simulink library "halout"  (R2021b)
settings: Solver=VariableStepAuto  StartTime=0.0  StopTime=10.0  RelTol=1e-3
undefined symbols (not defined in the file): C_TASK_5MS_S, FALSE, KHAL_CAN1FDAPS3E2E_flg, KHAL_CAN1FDAPS3TxReq_flg, KHAL_CAN1FDVCU2E2E_flg, KHAL_CAN1FDVCU2TxReq_flg, KHAL_CAN1FDVCU3E2E_flg, KHAL_CAN1FDVCU3TxReq_flg, KHAL_CAN1TxReq_flg, KHAL_CAN2TxReq_flg, KHAL_CAN3FDVCU1TxReq_flg, KHAL_CAN3FDVCU2E2E_flg, KHAL_CAN3FDVCU2TxReq_flg, KHAL_CAN3TxReq_flg, KHAL_CAN4FDVCU1E2E_flg, KHAL_CAN4FDVCU1TxReq_flg, KHAL_CAN4TxReq_flg, KHAL_CAN5TxReq_flg, ONE_INT, TRUE, ZERO_INT
libraries: FVT_lib x383, simulink x179
(part 7 of 20)

== system halout/HAL_OUT/CAN3/FD_THCM2_0x186 ==
  BSCP_outputs : Inport  OutDataTypeStr=Bus: BSCP_outputs
  BOUTP_outputs : Inport  Port=2  OutDataTypeStr=Bus: BOUTP_outputs
  ACSubMode : Subsystem
  APTCActFrRiPwr : Subsystem
  BatLoopActWtFlw : Subsystem
  CCUCbnPreACWkSts : Subsystem
  CCUCbnPreEstimdTi : Subsystem
  CCUCbnPreSts : Subsystem
  CCUHiVoltageReq : Subsystem
  CoolgFanActDuty : Subsystem
  DeiceModReq : Subsystem
  FDBlowerCmd : Subsystem
  FDCompCmd : Subsystem
  FDEWP1Cmd : Subsystem
  FDEWP2Cmd : Subsystem
  FDEWP3Cmd : Subsystem
  FDEXV1Cmd : Subsystem
  FDEXV2Cmd : Subsystem
  FDFWVCmd : Subsystem
  FDFrLeAPTCHeatPwrCmd : Subsystem
  FDFrRiAPTCHeatPwrCmd : Subsystem
  FDFrWPTCHeatPwrCmd : Subsystem
  FDRrAPTCHeatPwrCmd : Subsystem
  FDSOTXVCmd : Subsystem
  FDSOV1Cmd : Subsystem
  FDSOV2Cmd : Subsystem
  FDSOV3Cmd : Subsystem
  FDTWVCmd : Subsystem
  Ground{,1..6} (7 alike) : Ground
  bus_creator : BusCreator  Inputs=26  OutDataTypeStr=Bus: DT_CAN3_SG_FD_THCM2  NonVirtualBus=on
  bus_selector : BusSelector  OutputSignals=VOUTP_ACSubMode_enum
  bus_selector1 : BusSelector  OutputSignals=VOUTP_CoolgFanActDuty_pct
  bus_selector10 : BusSelector  OutputSignals=VOUTP_FDFrLeAPTCHeatPwrCmd_W
  bus_selector11 : BusSelector  OutputSignals=VOUTP_FDFrRiAPTCHeatPwrCmd_W
  bus_selector12 : BusSelector  OutputSignals=VOUTP_FDFrWPTCHeatPwrCmd_W
  bus_selector13 : BusSelector  OutputSignals=VOUTP_FDRrAPTCHeatPwrCmd_W
  bus_selector14 : BusSelector  OutputSignals=VOUTP_FDSOTXVCmd_flg
  bus_selector15 : BusSelector  OutputSignals=VOUTP_FDSOV1Cmd_flg
  bus_selector16 : BusSelector  OutputSignals=VOUTP_FDSOV2Cmd_flg
  bus_selector17 : BusSelector  OutputSignals=VOUTP_FDSOV3Cmd_flg
  bus_selector18 : BusSelector  OutputSignals=VOUTP_FDTWVCmd_pct
  bus_selector2 : BusSelector  OutputSignals=VOUTP_FDBlowerCmd_pct
  bus_selector3 : BusSelector  OutputSignals=VOUTP_FDCompCmd_rpm
  bus_selector4 : BusSelector  OutputSignals=VOUTP_FDEWP1Cmd_enum
  bus_selector5 : BusSelector  OutputSignals=VOUTP_FDEWP2Cmd_enum
  bus_selector6 : BusSelector  OutputSignals=VOUTP_FDEWP3Cmd_enum
  bus_selector7 : BusSelector  OutputSignals=VOUTP_FDEXV1Cmd_step
  bus_selector8 : BusSelector  OutputSignals=VOUTP_FDEXV2Cmd_step
  bus_selector9 : BusSelector  OutputSignals=VOUTP_FDFWVCmd_flg
  FD_THCM2 : Outport
  wires:
  BSCP_outputs/1 -> [BSCP_outputs]
  BOUTP_outputs/1 -> [BOUTP_outputs]
  [CAN3_ACSubMode] -> bus_creator/1  "CAN3_ACSubMode"
  [CAN3_APTC_ActFrRiPwr] -> bus_creator/2  "CAN3_APTC_ActFrRiPwr"
  [CAN3_BatLoopActWtFlw] -> bus_creator/3  "CAN3_BatLoopActWtFlw"
  [CAN3_CCU_CbnPreACWkSts] -> bus_creator/4  "CAN3_CCU_CbnPreACWkSts"
  [CAN3_CCU_CbnPreEstimdTi] -> bus_creator/5  "CAN3_CCU_CbnPreEstimdTi"
  [CAN3_CCU_CbnPreSts] -> bus_creator/6  "CAN3_CCU_CbnPreSts"
  [CAN3_CCU_HiVoltageReq] -> bus_creator/7  "CAN3_CCU_HiVoltageReq"
  [CAN3_CoolgFanActDuty] -> bus_creator/8  "CAN3_CoolgFanActDuty"
  [CAN3_DeiceModReq] -> bus_creator/9  "CAN3_DeiceModReq"
  [CAN3_FD_Blower_Cmd] -> bus_creator/10  "CAN3_FD_Blower_Cmd"
  [CAN3_FD_Comp_Cmd] -> bus_creator/11  "CAN3_FD_Comp_Cmd"
  [CAN3_FD_EWP1_Cmd] -> bus_creator/12  "CAN3_FD_EWP1_Cmd"
  [CAN3_FD_EWP2_Cmd] -> bus_creator/13  "CAN3_FD_EWP2_Cmd"
  [CAN3_FD_EWP3_Cmd] -> bus_creator/14  "CAN3_FD_EWP3_Cmd"
  [CAN3_FD_EXV1_Cmd] -> bus_creator/15  "CAN3_FD_EXV1_Cmd"
  [CAN3_FD_EXV2_Cmd] -> bus_creator/16  "CAN3_FD_EXV2_Cmd"
  [CAN3_FD_FWV_Cmd] -> bus_creator/17  "CAN3_FD_FWV_Cmd"
  [CAN3_FD_FrLeAPTCHeatPwr_Cmd] -> bus_creator/18  "CAN3_FD_FrLeAPTCHeatPwr_Cmd"
  [CAN3_FD_FrRiAPTCHeatPwr_Cmd] -> bus_creator/19  "CAN3_FD_FrRiAPTCHeatPwr_Cmd"
  [CAN3_FD_FrWPTCHeatPwr_Cmd] -> bus_creator/20  "CAN3_FD_FrWPTCHeatPwr_Cmd"
  [CAN3_FD_RrAPTCHeatPwr_Cmd] -> bus_creator/21  "CAN3_FD_RrAPTCHeatPwr_Cmd"
  [CAN3_FD_SOTXV_Cmd] -> bus_creator/22  "CAN3_FD_SOTXV_Cmd"
  [CAN3_FD_SOV1_Cmd] -> bus_creator/23  "CAN3_FD_SOV1_Cmd"
  [CAN3_FD_SOV2_Cmd] -> bus_creator/24  "CAN3_FD_SOV2_Cmd"
  [CAN3_FD_SOV3_Cmd] -> bus_creator/25  "CAN3_FD_SOV3_Cmd"
  [CAN3_FD_TWV_Cmd] -> bus_creator/26  "CAN3_FD_TWV_Cmd"
  bus_creator/1 -> FD_THCM2/1
  ACSubMode/1(CAN3_ACSubMode) -> [CAN3_ACSubMode]
  APTCActFrRiPwr/1(CAN3_APTC_ActFrRiPwr) -> [CAN3_APTC_ActFrRiPwr]
  BatLoopActWtFlw/1(CAN3_BatLoopActWtFlw) -> [CAN3_BatLoopActWtFlw]
  CCUCbnPreACWkSts/1(CAN3_CCU_CbnPreACWkSts) -> [CAN3_CCU_CbnPreACWkSts]
  CCUCbnPreEstimdTi/1(CAN3_CCU_CbnPreEstimdTi) -> [CAN3_CCU_CbnPreEstimdTi]
  CCUCbnPreSts/1(CAN3_CCU_CbnPreSts) -> [CAN3_CCU_CbnPreSts]
  CCUHiVoltageReq/1(CAN3_CCU_HiVoltageReq) -> [CAN3_CCU_HiVoltageReq]
  CoolgFanActDuty/1(CAN3_CoolgFanActDuty) -> [CAN3_CoolgFanActDuty]
  DeiceModReq/1(CAN3_DeiceModReq) -> [CAN3_DeiceModReq]
  FDBlowerCmd/1(CAN3_FD_Blower_Cmd) -> [CAN3_FD_Blower_Cmd]
  FDCompCmd/1(CAN3_FD_Comp_Cmd) -> [CAN3_FD_Comp_Cmd]
  FDEWP1Cmd/1(CAN3_FD_EWP1_Cmd) -> [CAN3_FD_EWP1_Cmd]
  FDEWP2Cmd/1(CAN3_FD_EWP2_Cmd) -> [CAN3_FD_EWP2_Cmd]
  FDEWP3Cmd/1(CAN3_FD_EWP3_Cmd) -> [CAN3_FD_EWP3_Cmd]
  FDEXV1Cmd/1(CAN3_FD_EXV1_Cmd) -> [CAN3_FD_EXV1_Cmd]
  FDEXV2Cmd/1(CAN3_FD_EXV2_Cmd) -> [CAN3_FD_EXV2_Cmd]
  FDFWVCmd/1(CAN3_FD_FWV_Cmd) -> [CAN3_FD_FWV_Cmd]
  FDFrLeAPTCHeatPwrCmd/1(CAN3_FD_FrLeAPTCHeatPwr_Cmd) -> [CAN3_FD_FrLeAPTCHeatPwr_Cmd]
  FDFrRiAPTCHeatPwrCmd/1(CAN3_FD_FrRiAPTCHeatPwr_Cmd) -> [CAN3_FD_FrRiAPTCHeatPwr_Cmd]
  FDFrWPTCHeatPwrCmd/1(CAN3_FD_FrWPTCHeatPwr_Cmd) -> [CAN3_FD_FrWPTCHeatPwr_Cmd]
  FDRrAPTCHeatPwrCmd/1(CAN3_FD_RrAPTCHeatPwr_Cmd) -> [CAN3_FD_RrAPTCHeatPwr_Cmd]
  FDSOTXVCmd/1(CAN3_FD_SOTXV_Cmd) -> [CAN3_FD_SOTXV_Cmd]
  FDSOV1Cmd/1(CAN3_FD_SOV1_Cmd) -> [CAN3_FD_SOV1_Cmd]
  FDSOV2Cmd/1(CAN3_FD_SOV2_Cmd) -> [CAN3_FD_SOV2_Cmd]
  FDSOV3Cmd/1(CAN3_FD_SOV3_Cmd) -> [CAN3_FD_SOV3_Cmd]
  FDTWVCmd/1(CAN3_FD_TWV_Cmd) -> [CAN3_FD_TWV_Cmd]
  bus_selector/1 -> ACSubMode/1(ACSubMode)  "<VOUTP_ACSubMode_enum>"
  [BOUTP_outputs] -> bus_selector/1
  Ground/1 -> APTCActFrRiPwr/1(APTCActFrRiPwr)
  Ground1/1 -> BatLoopActWtFlw/1(BatLoopActWtFlw)
  Ground2/1 -> CCUCbnPreACWkSts/1(CCUCbnPreACWkSts)
  Ground3/1 -> CCUCbnPreEstimdTi/1(CCUCbnPreEstimdTi)
  Ground4/1 -> CCUCbnPreSts/1(CCUCbnPreSts)
  Ground5/1 -> CCUHiVoltageReq/1(CCUHiVoltageReq)
  bus_selector1/1 -> CoolgFanActDuty/1(CoolgFanActDuty)  "<VOUTP_CoolgFanActDuty_pct>"
  [BOUTP_outputs] -> bus_selector1/1
  Ground6/1 -> DeiceModReq/1(DeiceModReq)
  bus_selector2/1 -> FDBlowerCmd/1(FDBlowerCmd)  "<VOUTP_FDBlowerCmd_pct>"
  [BOUTP_outputs] -> bus_selector2/1
  bus_selector3/1 -> FDCompCmd/1(FDCompCmd)  "<VOUTP_FDCompCmd_rpm>"
  [BOUTP_outputs] -> bus_selector3/1
  bus_selector4/1 -> FDEWP1Cmd/1(FDEWP1Cmd)  "<VOUTP_FDEWP1Cmd_enum>"
  [BOUTP_outputs] -> bus_selector4/1
  bus_selector5/1 -> FDEWP2Cmd/1(FDEWP2Cmd)  "<VOUTP_FDEWP2Cmd_enum>"
  [BOUTP_outputs] -> bus_selector5/1
  bus_selector6/1 -> FDEWP3Cmd/1(FDEWP3Cmd)  "<VOUTP_FDEWP3Cmd_enum>"
  [BOUTP_outputs] -> bus_selector6/1
  bus_selector7/1 -> FDEXV1Cmd/1(FDEXV1Cmd)  "<VOUTP_FDEXV1Cmd_step>"
  [BOUTP_outputs] -> bus_selector7/1
  bus_selector8/1 -> FDEXV2Cmd/1(FDEXV2Cmd)  "<VOUTP_FDEXV2Cmd_step>"
  [BOUTP_outputs] -> bus_selector8/1
  bus_selector9/1 -> FDFWVCmd/1(FDFWVCmd)  "<VOUTP_FDFWVCmd_flg>"
  [BOUTP_outputs] -> bus_selector9/1
  bus_selector10/1 -> FDFrLeAPTCHeatPwrCmd/1(FDFrLeAPTCHeatPwrCmd)  "<VOUTP_FDFrLeAPTCHeatPwrCmd_W>"
  [BOUTP_outputs] -> bus_selector10/1
  bus_selector11/1 -> FDFrRiAPTCHeatPwrCmd/1(FDFrRiAPTCHeatPwrCmd)  "<VOUTP_FDFrRiAPTCHeatPwrCmd_W>"
  [BOUTP_outputs] -> bus_selector11/1
  bus_selector12/1 -> FDFrWPTCHeatPwrCmd/1(FDFrWPTCHeatPwrCmd)  "<VOUTP_FDFrWPTCHeatPwrCmd_W>"
  [BOUTP_outputs] -> bus_selector12/1
  bus_selector13/1 -> FDRrAPTCHeatPwrCmd/1(FDRrAPTCHeatPwrCmd)  "<VOUTP_FDRrAPTCHeatPwrCmd_W>"
  [BOUTP_outputs] -> bus_selector13/1
  bus_selector14/1 -> FDSOTXVCmd/1(FDSOTXVCmd)  "<VOUTP_FDSOTXVCmd_flg>"
  [BOUTP_outputs] -> bus_selector14/1
  bus_selector15/1 -> FDSOV1Cmd/1(FDSOV1Cmd)  "<VOUTP_FDSOV1Cmd_flg>"
  [BOUTP_outputs] -> bus_selector15/1
  bus_selector16/1 -> FDSOV2Cmd/1(FDSOV2Cmd)  "<VOUTP_FDSOV2Cmd_flg>"
  [BOUTP_outputs] -> bus_selector16/1
  bus_selector17/1 -> FDSOV3Cmd/1(FDSOV3Cmd)  "<VOUTP_FDSOV3Cmd_flg>"
  [BOUTP_outputs] -> bus_selector17/1
  bus_selector18/1 -> FDTWVCmd/1(FDTWVCmd)  "<VOUTP_FDTWVCmd_pct>"
  [BOUTP_outputs] -> bus_selector18/1

== system halout/HAL_OUT/CAN3/FD_V2L1_0x374 ==
  BSCP_outputs : Inport  OutDataTypeStr=Bus: BSCP_outputs
  BOUTP_outputs : Inport  Port=2  OutDataTypeStr=Bus: BOUTP_outputs
  Ground : Ground
  ReqOBCV2LEna : Subsystem
  ReqV2LIVIPopup : Subsystem
  ReqV2LSwOn : Subsystem
  bus_creator : BusCreator  Inputs=3  OutDataTypeStr=Bus: DT_CAN3_SG_FD_V2L1  NonVirtualBus=on
  bus_selector : BusSelector  OutputSignals=VOUTP_ReqOBCV2LEna_enum
  bus_selector1 : BusSelector  OutputSignals=VOUTP_ReqV2LIVIPopup_enum
  FD_V2L1 : Outport
  wires:
  BSCP_outputs/1 -> [BSCP_outputs]
  BOUTP_outputs/1 -> [BOUTP_outputs]
  [CAN3_Req_OBCV2LEna] -> bus_creator/1  "CAN3_Req_OBCV2LEna"
  [CAN3_Req_V2LSwOn] -> bus_creator/2  "CAN3_Req_V2LSwOn"
  [CAN3_Req_V2L_IVI_Popup] -> bus_creator/3  "CAN3_Req_V2L_IVI_Popup"
  bus_creator/1 -> FD_V2L1/1
  ReqOBCV2LEna/1(CAN3_Req_OBCV2LEna) -> [CAN3_Req_OBCV2LEna]
  ReqV2LSwOn/1(CAN3_Req_V2LSwOn) -> [CAN3_Req_V2LSwOn]
  ReqV2LIVIPopup/1(CAN3_Req_V2L_IVI_Popup) -> [CAN3_Req_V2L_IVI_Popup]
  bus_selector/1 -> ReqOBCV2LEna/1(ReqOBCV2LEna)  "<VOUTP_ReqOBCV2LEna_enum>"
  [BOUTP_outputs] -> bus_selector/1
  Ground/1 -> ReqV2LSwOn/1(ReqV2LSwOn)
  bus_selector1/1 -> ReqV2LIVIPopup/1(ReqV2LIVIPopup)  "<VOUTP_ReqV2LIVIPopup_enum>"
  [BOUTP_outputs] -> bus_selector1/1

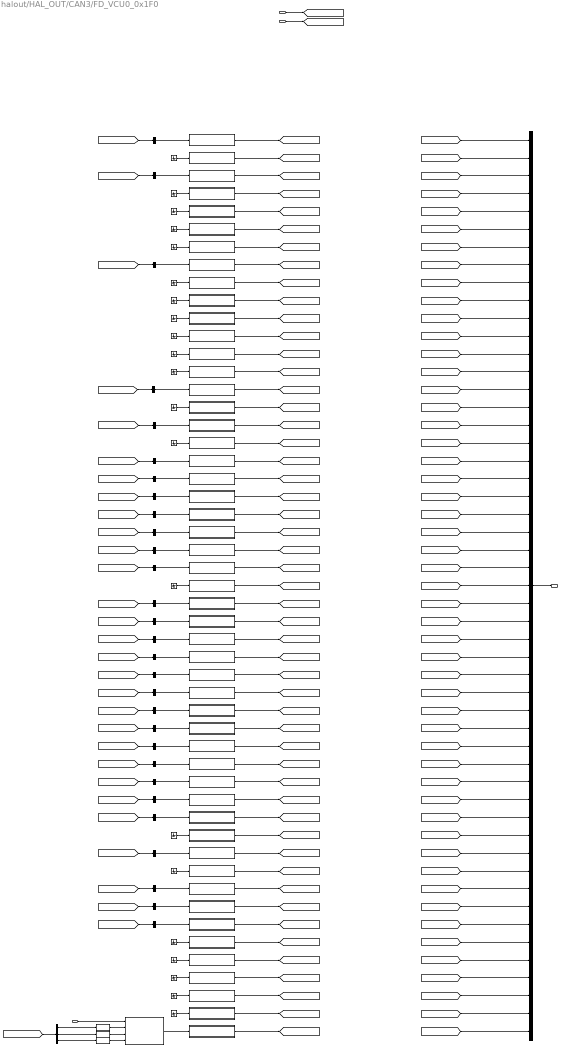
== system halout/HAL_OUT/CAN3/FD_VCU0_0x1F0 ==
  BSCP_outputs : Inport  OutDataTypeStr=Bus: BSCP_outputs
  BOUTP_outputs : Inport  Port=2  OutDataTypeStr=Bus: BOUTP_outputs
  s8_AcoreReadyToSleep : Inport  Port=3
  Data Type Conversion : DataTypeConversion  OutDataTypeStr=uint8
  Data Type Conversion1 : DataTypeConversion  OutDataTypeStr=uint8
  Data Type Conversion2 : DataTypeConversion  OutDataTypeStr=uint8
  EVCCAplusPwrUpReq : Subsystem
  FDADC12VDet : Subsystem
  FDADC12VDetAvg : Subsystem
  FDCVCUActMaxSlideRateSta : Subsystem
  FDCVCUAllowMovThdOTASta : Subsystem
  FDCVCUDTCCarouselSta : Subsystem
  FDCVCUForcePCmd : Subsystem
  FDCVCUPwrReqOTASta : Subsystem
  FDCVCURWDRDCActiveSta : Subsystem
  FDCVCURegenTqLimitEnSta : Subsystem
  FDCVCUSlideRegenLimTqSta : Subsystem
  FDCVCUVehActSpdSta : Subsystem
  FDCVCUVehMalfunLevelSta : Subsystem
  FDCVMCActStESCYawSta : Subsystem
  FDCVMCAntiSpdLimEnSta : Subsystem
  FDCVMCLongAccSta : Subsystem
  FrTqSource : Subsystem
  Ground{,1..10,12..21} (21 alike) : Ground
  HVRlyOpFail : Subsystem
  HVTHCMSysAvail : Subsystem
  LVBattChrgtimeAct : Subsystem
  LVBattVoltSta : Subsystem
  LVChrgHoldTAct : Subsystem
  LVSilentChrgLv : Subsystem
  LVSilentChrgReq : Subsystem
  LVSilentChrgSta : Subsystem
  MCUActDisFail : Subsystem
  PMMAllowECUSleep : Subsystem
  PowerDownFault : Subsystem
  PowerDownState : Subsystem
  PowerUpFault : Subsystem
  PowerUpState : Subsystem
  PwrDownReq : Subsystem
  PwrStaConstraint : Subsystem
  PwrStaONTOIVIPopReq : Subsystem
  PwrStaONTOIVIPopT : Subsystem
  PwrStaSelect : Subsystem
  PwrStaTOSta : Subsystem
  PwrUpReq : Subsystem
  RrTqSource : Subsystem
  SchedChgTOSta : Subsystem
  SilentChkAllowSleep : Subsystem
  Subsystem : Subsystem
  SysAllowReadySta : Subsystem
  SysPwrSta : Subsystem
  TCountSta : Subsystem
  TimerAllowSleep : Subsystem
  VCUBrkSWSta : Subsystem
  VCUFLDoorSta : Subsystem
  VCUFRDoorSta : Subsystem
  VCURLDoorSta : Subsystem
  VCURRDoorSta : Subsystem
  VehHVPwrAvail4THCM : Subsystem
  bus_creator : BusCreator  Inputs=51  OutDataTypeStr=Bus: DT_CAN3_SG_FD_VCU0  NonVirtualBus=on
  bus_selector : BusSelector  OutputSignals=VOUTP_EvccAplusPwrUpReq_flg
  bus_selector1 : BusSelector  OutputSignals=VOUTP_FDADC12VDetAvg_mV
  bus_selector10 : BusSelector  OutputSignals=VOUTP_LVSilentChrgSta_enum
  bus_selector11 : BusSelector  OutputSignals=VOUTP_PMMAllowECUSleep_flg
  bus_selector12 : BusSelector  OutputSignals=VOUTP_PowerDownFault_enum
  bus_selector13 : BusSelector  OutputSignals=VOUTP_PowerDownState_enum
  bus_selector14 : BusSelector  OutputSignals=VOUTP_PowerUpFault_enum
  bus_selector15 : BusSelector  OutputSignals=VOUTP_PowerUpState_enum
  bus_selector16 : BusSelector  OutputSignals=VOUTP_PwrDownReq_enum
  bus_selector17 : BusSelector  OutputSignals=VOUTP_PwrStaConstraint_enum
  bus_selector18 : BusSelector  OutputSignals=VOUTP_PwrStaONTOPopReq_flg
  bus_selector19 : BusSelector  OutputSignals=VOUTP_IVIPwrStaONTOPopT_s
  bus_selector2 : BusSelector  OutputSignals=VOUTP_PwrReq_OTA_enum
  bus_selector20 : BusSelector  OutputSignals=VOUTP_PwrStaSelect_enum
  bus_selector21 : BusSelector  OutputSignals=VOUTP_PwrStaTOSta_enum
  bus_selector22 : BusSelector  OutputSignals=VOUTP_PwrUpReq_enum
  bus_selector23 : BusSelector  OutputSignals=VOUTP_TqSourceRr_enum
  bus_selector24 : BusSelector  OutputSignals=VOUTP_SilentChkAllowSleep_flg
  bus_selector25 : BusSelector  OutputSignals=VOUTP_SysPowerMode_enum
  bus_selector26 : BusSelector  OutputSignals=VOUTP_TCountSta_enum
  bus_selector27 : BusSelector  OutputSignals=VOUTP_TimerAllowSleep_flg
  bus_selector28 : BusSelector  OutputSignals=VOUTP_CurrentNmState_enum,VOUTP_OTAPwrReqOFFChkSta_enum,VOUTP_OTAPwrReqStdChkSta_enum
  bus_selector29 : BusSelector  OutputSignals=VOUTP_ExtraMSACtrlSta_enum
  bus_selector3 : BusSelector  OutputSignals=VOUTP_TqSourceFr_enum
  bus_selector4 : BusSelector  OutputSignals=VOUTP_HVTHCMSysAvail_enum
  bus_selector5 : BusSelector  OutputSignals=VOUTP_LVBattChrgTimeCnt_s
  bus_selector6 : BusSelector  OutputSignals=VOUTP_LVBattVoltSta_enum
  bus_selector7 : BusSelector  OutputSignals=VOUTP_LVChrgHoldTtimer_s
  bus_selector8 : BusSelector  OutputSignals=VOUTP_LVSilentChrgLv_enum
  bus_selector9 : BusSelector  OutputSignals=VOUTP_LVSilentChrgReq_flg
  FD_VCU0 : Outport
  wires:
  BSCP_outputs/1 -> [BSCP_outputs]
  BOUTP_outputs/1 -> [BOUTP_outputs]
  [CAN3_EVCCAplusPwrUpReq] -> bus_creator/1  "CAN3_EVCCAplusPwrUpReq"
  [CAN3_FDADC12VDet] -> bus_creator/2  "CAN3_FDADC12VDet"
  [CAN3_FDADC12VDetAvg] -> bus_creator/3  "CAN3_FDADC12VDetAvg"
  [CAN3_FDC_VCU_ActMaxSlideRate_Sta] -> bus_creator/4  "CAN3_FDC_VCU_ActMaxSlideRate_Sta"
  [CAN3_FDC_VCU_AllowMovThd_OTA_Sta] -> bus_creator/5  "CAN3_FDC_VCU_AllowMovThd_OTA_Sta"
  [CAN3_FDC_VCU_DTCCarousel_Sta] -> bus_creator/6  "CAN3_FDC_VCU_DTCCarousel_Sta"
  [CAN3_FDC_VCU_ForceP_Cmd] -> bus_creator/7  "CAN3_FDC_VCU_ForceP_Cmd"
  [CAN3_FDC_VCU_PwrReq_OTA_Sta] -> bus_creator/8  "CAN3_FDC_VCU_PwrReq_OTA_Sta"
  [CAN3_FDC_VCU_RWDRDCActive_Sta] -> bus_creator/9  "CAN3_FDC_VCU_RWDRDCActive_Sta"
  [CAN3_FDC_VCU_RegenTqLimitEn_Sta] -> bus_creator/10  "CAN3_FDC_VCU_RegenTqLimitEn_Sta"
  [CAN3_FDC_VCU_SlideRegenLimTq_Sta] -> bus_creator/11  "CAN3_FDC_VCU_SlideRegenLimTq_Sta"
  [CAN3_FDC_VCU_VehActSpd_Sta] -> bus_creator/12  "CAN3_FDC_VCU_VehActSpd_Sta"
  [CAN3_FDC_VCU_VehMalfunLevel_Sta] -> bus_creator/13  "CAN3_FDC_VCU_VehMalfunLevel_Sta"
  [CAN3_FDC_VMC_ActStESCYaw_Sta] -> bus_creator/14  "CAN3_FDC_VMC_ActStESCYaw_Sta"
  [CAN3_FDC_VMC_AntiSpdLimEn_Sta] -> bus_creator/15  "CAN3_FDC_VMC_AntiSpdLimEn_Sta"
  [CAN3_FDC_VMC_LongAcc_Sta] -> bus_creator/16  "CAN3_FDC_VMC_LongAcc_Sta"
  [CAN3_Fr_TqSource] -> bus_creator/17  "CAN3_Fr_TqSource"
  [CAN3_HVRlyOpFail] -> bus_creator/18  "CAN3_HVRlyOpFail"
  [CAN3_HVTHCMSysAvail] -> bus_creator/19  "CAN3_HVTHCMSysAvail"
  [CAN3_LVBattChrgtimeAct] -> bus_creator/20  "CAN3_LVBattChrgtimeAct"
  [CAN3_LVBattVoltSta] -> bus_creator/21  "CAN3_LVBattVoltSta"
  [CAN3_LVChrgHoldTAct] -> bus_creator/22  "CAN3_LVChrgHoldTAct"
  [CAN3_LVSilentChrgLv] -> bus_creator/23  "CAN3_LVSilentChrgLv"
  [CAN3_LVSilentChrgReq] -> bus_creator/24  "CAN3_LVSilentChrgReq"
  [CAN3_LVSilentChrgSta] -> bus_creator/25  "CAN3_LVSilentChrgSta"
  [CAN3_MCUActDisFail] -> bus_creator/26  "CAN3_MCUActDisFail"
  [CAN3_PMMAllowECUSleep] -> bus_creator/27  "CAN3_PMMAllowECUSleep"
  [CAN3_PowerDownFault] -> bus_creator/28  "CAN3_PowerDownFault"
  [CAN3_PowerDownState] -> bus_creator/29  "CAN3_PowerDownState"
  [CAN3_PowerUpFault] -> bus_creator/30  "CAN3_PowerUpFault"
  [CAN3_PowerUpState] -> bus_creator/31  "CAN3_PowerUpState"
  [CAN3_PwrDownReq] -> bus_creator/32  "CAN3_PwrDownReq"
  [CAN3_PwrStaConstraint] -> bus_creator/33  "CAN3_PwrStaConstraint"
  [CAN3_PwrStaONTOIVIPopReq] -> bus_creator/34  "CAN3_PwrStaONTOIVIPopReq"
  [CAN3_PwrStaONTOIVIPopT] -> bus_creator/35  "CAN3_PwrStaONTOIVIPopT"
  [CAN3_PwrStaSelect] -> bus_creator/36  "CAN3_PwrStaSelect"
  [CAN3_PwrStaTOSta] -> bus_creator/37  "CAN3_PwrStaTOSta"
  [CAN3_PwrUpReq] -> bus_creator/38  "CAN3_PwrUpReq"
  [CAN3_Rr_TqSource] -> bus_creator/39  "CAN3_Rr_TqSource"
  [CAN3_SchedChgTOSta] -> bus_creator/40  "CAN3_SchedChgTOSta"
  [CAN3_SilentChkAllowSleep] -> bus_creator/41  "CAN3_SilentChkAllowSleep"
  [CAN3_SysAllowReadySta] -> bus_creator/42  "CAN3_SysAllowReadySta"
  [CAN3_SysPwrSta] -> bus_creator/43  "CAN3_SysPwrSta"
  [CAN3_TCountSta] -> bus_creator/44  "CAN3_TCountSta"
  [CAN3_TimerAllowSleep] -> bus_creator/45  "CAN3_TimerAllowSleep"
  [CAN3_VCUBrkSWSta] -> bus_creator/46  "CAN3_VCUBrkSWSta"
  [CAN3_VCUFLDoorSta] -> bus_creator/47  "CAN3_VCUFLDoorSta"
  [CAN3_VCUFRDoorSta] -> bus_creator/48  "CAN3_VCUFRDoorSta"
  [CAN3_VCURLDoorSta] -> bus_creator/49  "CAN3_VCURLDoorSta"
  [CAN3_VCURRDoorSta] -> bus_creator/50  "CAN3_VCURRDoorSta"
  [CAN3_VehHVPwrAvail4THCM] -> bus_creator/51  "CAN3_VehHVPwrAvail4THCM"
  bus_creator/1 -> FD_VCU0/1
  EVCCAplusPwrUpReq/1(CAN3_EVCCAplusPwrUpReq) -> [CAN3_EVCCAplusPwrUpReq]
  FDADC12VDet/1(CAN3_FDADC12VDet) -> [CAN3_FDADC12VDet]
  FDADC12VDetAvg/1(CAN3_FDADC12VDetAvg) -> [CAN3_FDADC12VDetAvg]
  FDCVCUActMaxSlideRateSta/1(CAN3_FDC_VCU_ActMaxSlideRate_Sta) -> [CAN3_FDC_VCU_ActMaxSlideRate_Sta]
  FDCVCUAllowMovThdOTASta/1(CAN3_FDC_VCU_AllowMovThd_OTA_Sta) -> [CAN3_FDC_VCU_AllowMovThd_OTA_Sta]
  FDCVCUDTCCarouselSta/1(CAN3_FDC_VCU_DTCCarousel_Sta) -> [CAN3_FDC_VCU_DTCCarousel_Sta]
  FDCVCUForcePCmd/1(CAN3_FDC_VCU_ForceP_Cmd) -> [CAN3_FDC_VCU_ForceP_Cmd]
  FDCVCUPwrReqOTASta/1(CAN3_FDC_VCU_PwrReq_OTA_Sta) -> [CAN3_FDC_VCU_PwrReq_OTA_Sta]
  FDCVCURWDRDCActiveSta/1(CAN3_FDC_VCU_RWDRDCActive_Sta) -> [CAN3_FDC_VCU_RWDRDCActive_Sta]
  FDCVCURegenTqLimitEnSta/1(CAN3_FDC_VCU_RegenTqLimitEn_Sta) -> [CAN3_FDC_VCU_RegenTqLimitEn_Sta]
  FDCVCUSlideRegenLimTqSta/1(CAN3_FDC_VCU_SlideRegenLimTq_Sta) -> [CAN3_FDC_VCU_SlideRegenLimTq_Sta]
  FDCVCUVehActSpdSta/1(CAN3_FDC_VCU_VehActSpd_Sta) -> [CAN3_FDC_VCU_VehActSpd_Sta]
  FDCVCUVehMalfunLevelSta/1(CAN3_FDC_VCU_VehMalfunLevel_Sta) -> [CAN3_FDC_VCU_VehMalfunLevel_Sta]
  FDCVMCActStESCYawSta/1(CAN3_FDC_VMC_ActStESCYaw_Sta) -> [CAN3_FDC_VMC_ActStESCYaw_Sta]
  FDCVMCAntiSpdLimEnSta/1(CAN3_FDC_VMC_AntiSpdLimEn_Sta) -> [CAN3_FDC_VMC_AntiSpdLimEn_Sta]
  FDCVMCLongAccSta/1(CAN3_FDC_VMC_LongAcc_Sta) -> [CAN3_FDC_VMC_LongAcc_Sta]
  FrTqSource/1(CAN3_Fr_TqSource) -> [CAN3_Fr_TqSource]
  HVRlyOpFail/1(CAN3_HVRlyOpFail) -> [CAN3_HVRlyOpFail]
  HVTHCMSysAvail/1(CAN3_HVTHCMSysAvail) -> [CAN3_HVTHCMSysAvail]
  LVBattChrgtimeAct/1(CAN3_LVBattChrgtimeAct) -> [CAN3_LVBattChrgtimeAct]
  LVBattVoltSta/1(CAN3_LVBattVoltSta) -> [CAN3_LVBattVoltSta]
  LVChrgHoldTAct/1(CAN3_LVChrgHoldTAct) -> [CAN3_LVChrgHoldTAct]
  LVSilentChrgLv/1(CAN3_LVSilentChrgLv) -> [CAN3_LVSilentChrgLv]
  LVSilentChrgReq/1(CAN3_LVSilentChrgReq) -> [CAN3_LVSilentChrgReq]
  LVSilentChrgSta/1(CAN3_LVSilentChrgSta) -> [CAN3_LVSilentChrgSta]
  MCUActDisFail/1(CAN3_MCUActDisFail) -> [CAN3_MCUActDisFail]
  PMMAllowECUSleep/1(CAN3_PMMAllowECUSleep) -> [CAN3_PMMAllowECUSleep]
  PowerDownFault/1(CAN3_PowerDownFault) -> [CAN3_PowerDownFault]
  PowerDownState/1(CAN3_PowerDownState) -> [CAN3_PowerDownState]
  PowerUpFault/1(CAN3_PowerUpFault) -> [CAN3_PowerUpFault]
  PowerUpState/1(CAN3_PowerUpState) -> [CAN3_PowerUpState]
  PwrDownReq/1(CAN3_PwrDownReq) -> [CAN3_PwrDownReq]
  PwrStaConstraint/1(CAN3_PwrStaConstraint) -> [CAN3_PwrStaConstraint]
  PwrStaONTOIVIPopReq/1(CAN3_PwrStaONTOIVIPopReq) -> [CAN3_PwrStaONTOIVIPopReq]
  PwrStaONTOIVIPopT/1(CAN3_PwrStaONTOIVIPopT) -> [CAN3_PwrStaONTOIVIPopT]
  PwrStaSelect/1(CAN3_PwrStaSelect) -> [CAN3_PwrStaSelect]
  PwrStaTOSta/1(CAN3_PwrStaTOSta) -> [CAN3_PwrStaTOSta]
  PwrUpReq/1(CAN3_PwrUpReq) -> [CAN3_PwrUpReq]
  RrTqSource/1(CAN3_Rr_TqSource) -> [CAN3_Rr_TqSource]
  SchedChgTOSta/1(CAN3_SchedChgTOSta) -> [CAN3_SchedChgTOSta]
  SilentChkAllowSleep/1(CAN3_SilentChkAllowSleep) -> [CAN3_SilentChkAllowSleep]
  SysAllowReadySta/1(CAN3_SysAllowReadySta) -> [CAN3_SysAllowReadySta]
  SysPwrSta/1(CAN3_SysPwrSta) -> [CAN3_SysPwrSta]
  TCountSta/1(CAN3_TCountSta) -> [CAN3_TCountSta]
  TimerAllowSleep/1(CAN3_TimerAllowSleep) -> [CAN3_TimerAllowSleep]
  VCUBrkSWSta/1(CAN3_VCUBrkSWSta) -> [CAN3_VCUBrkSWSta]
  VCUFLDoorSta/1(CAN3_VCUFLDoorSta) -> [CAN3_VCUFLDoorSta]
  VCUFRDoorSta/1(CAN3_VCUFRDoorSta) -> [CAN3_VCUFRDoorSta]
  VCURLDoorSta/1(CAN3_VCURLDoorSta) -> [CAN3_VCURLDoorSta]
  VCURRDoorSta/1(CAN3_VCURRDoorSta) -> [CAN3_VCURRDoorSta]
  VehHVPwrAvail4THCM/1(CAN3_VehHVPwrAvail4THCM) -> [CAN3_VehHVPwrAvail4THCM]
  bus_selector/1 -> EVCCAplusPwrUpReq/1(EVCCAplusPwrUpReq)  "<VOUTP_EvccAplusPwrUpReq_flg>"
  [BOUTP_outputs] -> bus_selector/1
  Ground/1 -> FDADC12VDet/1(FDADC12VDet)
  bus_selector1/1 -> FDADC12VDetAvg/1(FDADC12VDetAvg)  "<VOUTP_FDADC12VDetAvg_mV>"
  [BOUTP_outputs] -> bus_selector1/1
  Ground1/1 -> FDCVCUActMaxSlideRateSta/1(FDCVCUActMaxSlideRateSta)
  Ground2/1 -> FDCVCUAllowMovThdOTASta/1(FDCVCUAllowMovThdOTASta)
  Ground3/1 -> FDCVCUDTCCarouselSta/1(FDCVCUDTCCarouselSta)
  Ground4/1 -> FDCVCUForcePCmd/1(FDCVCUForcePCmd)
  bus_selector2/1 -> FDCVCUPwrReqOTASta/1(FDCVCUPwrReqOTASta)  "<VOUTP_PwrReq_OTA_enum>"
  [BOUTP_outputs] -> bus_selector2/1
  Ground5/1 -> FDCVCURWDRDCActiveSta/1(FDCVCURWDRDCActiveSta)
  Ground6/1 -> FDCVCURegenTqLimitEnSta/1(FDCVCURegenTqLimitEnSta)
  Ground7/1 -> FDCVCUSlideRegenLimTqSta/1(FDCVCUSlideRegenLimTqSta)
  Ground8/1 -> FDCVCUVehActSpdSta/1(FDCVCUVehActSpdSta)
  Ground9/1 -> FDCVCUVehMalfunLevelSta/1(FDCVCUVehMalfunLevelSta)
  Ground10/1 -> FDCVMCActStESCYawSta/1(FDCVMCActStESCYawSta)
  Ground12/1 -> FDCVMCLongAccSta/1(FDCVMCLongAccSta)
  bus_selector3/1 -> FrTqSource/1(FrTqSource)  "<VOUTP_TqSourceFr_enum>"
  [BOUTP_outputs] -> bus_selector3/1
  Ground13/1 -> HVRlyOpFail/1(HVRlyOpFail)
  bus_selector4/1 -> HVTHCMSysAvail/1(HVTHCMSysAvail)  "<VOUTP_HVTHCMSysAvail_enum>"
  [BOUTP_outputs] -> bus_selector4/1
  bus_selector5/1 -> LVBattChrgtimeAct/1(LVBattChrgtimeAct)  "<VOUTP_LVBattChrgTimeCnt_s>"
  [BOUTP_outputs] -> bus_selector5/1
  bus_selector6/1 -> LVBattVoltSta/1(LVBattVoltSta)  "<VOUTP_LVBattVoltSta_enum>"
  [BOUTP_outputs] -> bus_selector6/1
  bus_selector7/1 -> LVChrgHoldTAct/1(LVChrgHoldTAct)  "<VOUTP_LVChrgHoldTtimer_s>"
  [BOUTP_outputs] -> bus_selector7/1
  bus_selector8/1 -> LVSilentChrgLv/1(LVSilentChrgLv)  "<VOUTP_LVSilentChrgLv_enum>"
  [BOUTP_outputs] -> bus_selector8/1
  bus_selector9/1 -> LVSilentChrgReq/1(LVSilentChrgReq)  "<VOUTP_LVSilentChrgReq_flg>"
  [BOUTP_outputs] -> bus_selector9/1
  bus_selector10/1 -> LVSilentChrgSta/1(LVSilentChrgSta)  "<VOUTP_LVSilentChrgSta_enum>"
  [BOUTP_outputs] -> bus_selector10/1
  Ground14/1 -> MCUActDisFail/1(MCUActDisFail)
  bus_selector11/1 -> PMMAllowECUSleep/1(PMMAllowECUSleep)  "<VOUTP_PMMAllowECUSleep_flg>"
  [BOUTP_outputs] -> bus_selector11/1
  bus_selector12/1 -> PowerDownFault/1(PowerDownFault)  "<VOUTP_PowerDownFault_enum>"
  [BOUTP_outputs] -> bus_selector12/1
  bus_selector13/1 -> PowerDownState/1(PowerDownState)  "<VOUTP_PowerDownState_enum>"
  [BOUTP_outputs] -> bus_selector13/1
  bus_selector14/1 -> PowerUpFault/1(PowerUpFault)  "<VOUTP_PowerUpFault_enum>"
  [BOUTP_outputs] -> bus_selector14/1
  bus_selector15/1 -> PowerUpState/1(PowerUpState)  "<VOUTP_PowerUpState_enum>"
  [BOUTP_outputs] -> bus_selector15/1
  bus_selector16/1 -> PwrDownReq/1(PwrDownReq)  "<VOUTP_PwrDownReq_enum>"
  [BOUTP_outputs] -> bus_selector16/1
  bus_selector17/1 -> PwrStaConstraint/1(PwrStaConstraint)  "<VOUTP_PwrStaConstraint_enum>"
  [BOUTP_outputs] -> bus_selector17/1
  bus_selector18/1 -> PwrStaONTOIVIPopReq/1(PwrStaONTOIVIPopReq)  "<VOUTP_PwrStaONTOPopReq_flg>"
  [BOUTP_outputs] -> bus_selector18/1
  bus_selector19/1 -> PwrStaONTOIVIPopT/1(PwrStaONTOIVIPopT)  "<VOUTP_IVIPwrStaONTOPopT_s>"
  [BOUTP_outputs] -> bus_selector19/1
  bus_selector20/1 -> PwrStaSelect/1(PwrStaSelect)  "<VOUTP_PwrStaSelect_enum>"
  [BOUTP_outputs] -> bus_selector20/1
  bus_selector21/1 -> PwrStaTOSta/1(PwrStaTOSta)  "<VOUTP_PwrStaTOSta_enum>"
  [BOUTP_outputs] -> bus_selector21/1
  bus_selector22/1 -> PwrUpReq/1(PwrUpReq)  "<VOUTP_PwrUpReq_enum>"
  [BOUTP_outputs] -> bus_selector22/1
  bus_selector23/1 -> RrTqSource/1(RrTqSource)  "<VOUTP_TqSourceRr_enum>"
  [BOUTP_outputs] -> bus_selector23/1
  Ground15/1 -> SchedChgTOSta/1(SchedChgTOSta)
  bus_selector24/1 -> SilentChkAllowSleep/1(SilentChkAllowSleep)  "<VOUTP_SilentChkAllowSleep_flg>"
  [BOUTP_outputs] -> bus_selector24/1
  Ground16/1 -> SysAllowReadySta/1(SysAllowReadySta)
  bus_selector25/1 -> SysPwrSta/1(SysPwrSta)  "<VOUTP_SysPowerMode_enum>"
  [BOUTP_outputs] -> bus_selector25/1
  bus_selector26/1 -> TCountSta/1(TCountSta)  "<VOUTP_TCountSta_enum>"
  [BOUTP_outputs] -> bus_selector26/1
  bus_selector27/1 -> TimerAllowSleep/1(TimerAllowSleep)  "<VOUTP_TimerAllowSleep_flg>"
  [BOUTP_outputs] -> bus_selector27/1
  Ground17/1 -> VCUBrkSWSta/1(VCUBrkSWSta)
  Ground18/1 -> VCUFLDoorSta/1(VCUFLDoorSta)
  Ground19/1 -> VCUFRDoorSta/1(VCUFRDoorSta)
  Ground20/1 -> VCURLDoorSta/1(VCURLDoorSta)
  Ground21/1 -> VCURRDoorSta/1(VCURRDoorSta)
  bus_selector28/1 -> Data Type Conversion/1  "<VOUTP_CurrentNmState_enum>"
  s8_AcoreReadyToSleep/1 -> Subsystem/1(s8_AcoreReadyToSleep)
  bus_selector28/2 -> Data Type Conversion1/1  "<VOUTP_OTAPwrReqOFFChkSta_enum>"
  Data Type Conversion1/1 -> Subsystem/3(VOUTP_OTAPwrReqOFFChkSta_enum)
  Data Type Conversion2/1 -> Subsystem/4(VOUTP_OTAPwrReqStdChkSta_enum)
  bus_selector28/3 -> Data Type Conversion2/1  "<VOUTP_OTAPwrReqStdChkSta_enum>"
  [BOUTP_outputs] -> bus_selector28/1
  Data Type Conversion/1 -> Subsystem/2(VOUTP_CurrentNmState_enum)
  Subsystem/1(VehHVPwrAvail4THCM) -> VehHVPwrAvail4THCM/1(VehHVPwrAvail4THCM)
  [BOUTP_outputs] -> bus_selector29/1
  bus_selector29/1 -> FDCVMCAntiSpdLimEnSta/1(FDCVMCAntiSpdLimEnSta)  "<VOUTP_ExtraMSACtrlSta_enum>"

== system halout/HAL_OUT/CAN3/FD_VCU1_0x116 ==
  BSCP_outputs : Inport  OutDataTypeStr=Bus: BSCP_outputs
  BOUTP_outputs : Inport  Port=2  OutDataTypeStr=Bus: BOUTP_outputs
  ActiveDischReq : Subsystem
  CSVCU1 : Subsystem
  CoastDwModeStaChk : Subsystem
  DCDCEnaReq : Subsystem
  DCDCVoltSetpoint : Subsystem
  DemoModeStaChk : Subsystem
  DrSeatSta : Subsystem
  DynoModeStaChk : Subsystem
  FrActvDmpDisabReq : Subsystem
  FrMCUEnaReq : Subsystem
  Ground{,1..5} (6 alike) : Ground
  HVBatCnctReq : Subsystem
  HVSysReadyToCharge : Subsystem
  LVChrgFuncStaChk : Subsystem
  MSACrlSta : Subsystem
  PrkReq : Subsystem
  PwrSta : Subsystem
  RCVCU1 : Subsystem
  RrActvDmpDisabReq : Subsystem
  RrMCUEnaReq : Subsystem
  ShiftGearPosn : Subsystem
  bus_creator : BusCreator  Inputs=20  OutDataTypeStr=Bus: DT_CAN3_SG_FD_VCU1  NonVirtualBus=on
  bus_selector : BusSelector  OutputSignals=VOUTP_ActiveDischargeReq_flg
  bus_selector1 : BusSelector  OutputSignals=VOUTP_DCDCEnaReq_flg
  bus_selector10 : BusSelector  OutputSignals=VOUTP_PowerSta_enum
  bus_selector11 : BusSelector  OutputSignals=VOUTP_RrActvDmpDisabReq_flg
  bus_selector12 : BusSelector  OutputSignals=VOUTP_RrMCUEnaReq_flg
  bus_selector13 : BusSelector  OutputSignals=VOUTP_ShiftGearPosn_enum
  bus_selector2 : BusSelector  OutputSignals=VOUTP_DCDCVoltSetpoint_V
  bus_selector3 : BusSelector  OutputSignals=VOUTP_DrSeatSta_enum
  bus_selector4 : BusSelector  OutputSignals=VOUTP_FrActvDmpDisabReq_flg
  bus_selector5 : BusSelector  OutputSignals=VOUTP_FrMCUEnaReq_flg
  bus_selector6 : BusSelector  OutputSignals=VOUTP_HVBatCnctReq_flg
  bus_selector7 : BusSelector  OutputSignals=VOUTP_HVSysReadyToCharge_enum
  bus_selector8 : BusSelector  OutputSignals=VOUTP_MSACtrlSta_enum
  bus_selector9 : BusSelector  OutputSignals=VOUTP_ActParkRequest_flg
  FD_VCU1 : Outport
  wires:
  BSCP_outputs/1 -> [BSCP_outputs]
  BOUTP_outputs/1 -> [BOUTP_outputs]
  [CAN3_ActiveDischReq] -> bus_creator/1  "CAN3_ActiveDischReq"
  [CAN3_CS_VCU1] -> bus_creator/2  "CAN3_CS_VCU1"
  [CAN3_CoastDwModeStaChk] -> bus_creator/3  "CAN3_CoastDwModeStaChk"
  [CAN3_DCDCEnaReq] -> bus_creator/4  "CAN3_DCDCEnaReq"
  [CAN3_DCDCVoltSetpoint] -> bus_creator/5  "CAN3_DCDCVoltSetpoint"
  [CAN3_DemoModeStaChk] -> bus_creator/6  "CAN3_DemoModeStaChk"
  [CAN3_Dr_SeatSta] -> bus_creator/7  "CAN3_Dr_SeatSta"
  [CAN3_DynoModeStaChk] -> bus_creator/8  "CAN3_DynoModeStaChk"
  [CAN3_Fr_ActvDmpDisabReq] -> bus_creator/9  "CAN3_Fr_ActvDmpDisabReq"
  [CAN3_Fr_MCUEnaReq] -> bus_creator/10  "CAN3_Fr_MCUEnaReq"
  [CAN3_HVBatCnctReq] -> bus_creator/11  "CAN3_HVBatCnctReq"
  [CAN3_HVSysReadyToCharge] -> bus_creator/12  "CAN3_HVSysReadyToCharge"
  [CAN3_LVChrgFuncStaChk] -> bus_creator/13  "CAN3_LVChrgFuncStaChk"
  [CAN3_MSA_Crl_Sta] -> bus_creator/14  "CAN3_MSA_Crl_Sta"
  [CAN3_PrkReq] -> bus_creator/15  "CAN3_PrkReq"
  [CAN3_PwrSta] -> bus_creator/16  "CAN3_PwrSta"
  [CAN3_RC_VCU1] -> bus_creator/17  "CAN3_RC_VCU1"
  [CAN3_Rr_ActvDmpDisabReq] -> bus_creator/18  "CAN3_Rr_ActvDmpDisabReq"
  [CAN3_Rr_MCUEnaReq] -> bus_creator/19  "CAN3_Rr_MCUEnaReq"
  [CAN3_ShiftGearPosn] -> bus_creator/20  "CAN3_ShiftGearPosn"
  bus_creator/1 -> FD_VCU1/1
  ActiveDischReq/1(CAN3_ActiveDischReq) -> [CAN3_ActiveDischReq]
  CSVCU1/1(CAN3_CS_VCU1) -> [CAN3_CS_VCU1]
  CoastDwModeStaChk/1(CAN3_CoastDwModeStaChk) -> [CAN3_CoastDwModeStaChk]
  DCDCEnaReq/1(CAN3_DCDCEnaReq) -> [CAN3_DCDCEnaReq]
  DCDCVoltSetpoint/1(CAN3_DCDCVoltSetpoint) -> [CAN3_DCDCVoltSetpoint]
  DemoModeStaChk/1(CAN3_DemoModeStaChk) -> [CAN3_DemoModeStaChk]
  DrSeatSta/1(CAN3_Dr_SeatSta) -> [CAN3_Dr_SeatSta]
  DynoModeStaChk/1(CAN3_DynoModeStaChk) -> [CAN3_DynoModeStaChk]
  FrActvDmpDisabReq/1(CAN3_Fr_ActvDmpDisabReq) -> [CAN3_Fr_ActvDmpDisabReq]
  FrMCUEnaReq/1(CAN3_Fr_MCUEnaReq) -> [CAN3_Fr_MCUEnaReq]
  HVBatCnctReq/1(CAN3_HVBatCnctReq) -> [CAN3_HVBatCnctReq]
  HVSysReadyToCharge/1(CAN3_HVSysReadyToCharge) -> [CAN3_HVSysReadyToCharge]
  LVChrgFuncStaChk/1(CAN3_LVChrgFuncStaChk) -> [CAN3_LVChrgFuncStaChk]
  MSACrlSta/1(CAN3_MSA_Crl_Sta) -> [CAN3_MSA_Crl_Sta]
  PrkReq/1(CAN3_PrkReq) -> [CAN3_PrkReq]
  PwrSta/1(CAN3_PwrSta) -> [CAN3_PwrSta]
  RCVCU1/1(CAN3_RC_VCU1) -> [CAN3_RC_VCU1]
  RrActvDmpDisabReq/1(CAN3_Rr_ActvDmpDisabReq) -> [CAN3_Rr_ActvDmpDisabReq]
  RrMCUEnaReq/1(CAN3_Rr_MCUEnaReq) -> [CAN3_Rr_MCUEnaReq]
  ShiftGearPosn/1(CAN3_ShiftGearPosn) -> [CAN3_ShiftGearPosn]
  bus_selector/1 -> ActiveDischReq/1(ActiveDischReq)  "<VOUTP_ActiveDischargeReq_flg>"
  [BOUTP_outputs] -> bus_selector/1
  Ground/1 -> CSVCU1/1(CSVCU1)
  Ground1/1 -> CoastDwModeStaChk/1(CoastDwModeStaChk)
  bus_selector1/1 -> DCDCEnaReq/1(DCDCEnaReq)  "<VOUTP_DCDCEnaReq_flg>"
  [BOUTP_outputs] -> bus_selector1/1
  bus_selector2/1 -> DCDCVoltSetpoint/1(DCDCVoltSetpoint)  "<VOUTP_DCDCVoltSetpoint_V>"
  [BOUTP_outputs] -> bus_selector2/1
  Ground2/1 -> DemoModeStaChk/1(DemoModeStaChk)
  bus_selector3/1 -> DrSeatSta/1(DrSeatSta)  "<VOUTP_DrSeatSta_enum>"
  [BOUTP_outputs] -> bus_selector3/1
  Ground3/1 -> DynoModeStaChk/1(DynoModeStaChk)
  bus_selector4/1 -> FrActvDmpDisabReq/1(FrActvDmpDisabReq)  "<VOUTP_FrActvDmpDisabReq_flg>"
  [BOUTP_outputs] -> bus_selector4/1
  bus_selector5/1 -> FrMCUEnaReq/1(FrMCUEnaReq)  "<VOUTP_FrMCUEnaReq_flg>"
  [BOUTP_outputs] -> bus_selector5/1
  bus_selector6/1 -> HVBatCnctReq/1(HVBatCnctReq)  "<VOUTP_HVBatCnctReq_flg>"
  [BOUTP_outputs] -> bus_selector6/1
  bus_selector7/1 -> HVSysReadyToCharge/1(HVSysReadyToCharge)  "<VOUTP_HVSysReadyToCharge_enum>"
  [BOUTP_outputs] -> bus_selector7/1
  Ground4/1 -> LVChrgFuncStaChk/1(LVChrgFuncStaChk)
  bus_selector8/1 -> MSACrlSta/1(MSACrlSta)  "<VOUTP_MSACtrlSta_enum>"
  [BOUTP_outputs] -> bus_selector8/1
  bus_selector9/1 -> PrkReq/1(PrkReq)  "<VOUTP_ActParkRequest_flg>"
  [BOUTP_outputs] -> bus_selector9/1
  bus_selector10/1 -> PwrSta/1(PwrSta)  "<VOUTP_PowerSta_enum>"
  [BOUTP_outputs] -> bus_selector10/1
  Ground5/1 -> RCVCU1/1(RCVCU1)
  bus_selector11/1 -> RrActvDmpDisabReq/1(RrActvDmpDisabReq)  "<VOUTP_RrActvDmpDisabReq_flg>"
  [BOUTP_outputs] -> bus_selector11/1
  bus_selector12/1 -> RrMCUEnaReq/1(RrMCUEnaReq)  "<VOUTP_RrMCUEnaReq_flg>"
  [BOUTP_outputs] -> bus_selector12/1
  bus_selector13/1 -> ShiftGearPosn/1(ShiftGearPosn)  "<VOUTP_ShiftGearPosn_enum>"
  [BOUTP_outputs] -> bus_selector13/1

== system halout/HAL_OUT/CAN3/FD_VCU1_Tx ==
  TxReq : Inport
  BSCP_outputs : Inport  Port=2  OutDataTypeStr=Bus: BSCP_outputs
  BOUTP_outputs : Inport  Port=3  OutDataTypeStr=Bus: BOUTP_outputs
  Chart1 : Stateflow chart  TreatAsAtomicUnit=on
  Constant : Constant  Value=C_TASK_5MS_S
  Constant3 : Constant  Value=CycleTime
  Data Type Conversion : DataTypeConversion  OutDataTypeStr=uint16
  Data Type Conversion1 : DataTypeConversion  OutDataTypeStr=uint8
  Divide : Product  Inputs=*/
  Gain : Gain  Gain=0.001
  Ground{,1..6} (7 alike) : Ground
  OR : Logic  Operator=OR  Inputs=20  AllPortsSameDT=off  OutDataTypeStr=boolean
  bus_selector : BusSelector  OutputSignals=VOUTP_ActiveDischargeReq_flg
  bus_selector1 : BusSelector  OutputSignals=VOUTP_DCDCEnaReq_flg
  bus_selector10 : BusSelector  OutputSignals=VOUTP_RrActvDmpDisabReq_flg
  bus_selector11 : BusSelector  OutputSignals=VOUTP_RrMCUEnaReq_flg
  bus_selector12 : BusSelector  OutputSignals=VOUTP_ShiftGearPosn_enum
  bus_selector2 : BusSelector  OutputSignals=VOUTP_DCDCVoltSetpoint_V
  bus_selector3 : BusSelector  OutputSignals=VOUTP_FrActvDmpDisabReq_flg
  bus_selector4 : BusSelector  OutputSignals=VOUTP_FrMCUEnaReq_flg
  bus_selector5 : BusSelector  OutputSignals=VOUTP_HVBatCnctReq_flg
  bus_selector6 : BusSelector  OutputSignals=VOUTP_HVSysReadyToCharge_enum
  bus_selector7 : BusSelector  OutputSignals=VOUTP_MSACtrlSta_enum
  bus_selector8 : BusSelector  OutputSignals=VOUTP_ActParkRequest_flg
  bus_selector9 : BusSelector  OutputSignals=VOUTP_PowerSta_enum
  convert_out : FVT_lib/hal/convert_out  gain=0.0235  offset=12
  detect_change{,1..12} (13 alike) : simulink/Logic and Bit Operations/Detect Change  vinit=0  OutDataTypeStr=boolean
  TxTrigger : Outport
  wires:
  Data Type Conversion/1 -> Chart1/3(CycleCnt)
  TxReq/1 -> Chart1/1(TxReq)
  [EventReq_flg] -> Chart1/2(EventReq)
  Constant/1 -> Divide/2
  Divide/1 -> Data Type Conversion/1
  Chart1/1(TxTrigger) -> TxTrigger/1
  Gain/1 -> Divide/1
  Constant3/1 -> Gain/1
  BSCP_outputs/1 -> [BSCP_outputs]
  BOUTP_outputs/1 -> [BOUTP_outputs]
  OR/1 -> [EventReq_flg]
  detect_change/1 -> OR/1
  bus_selector/1 -> detect_change/1  "<VOUTP_ActiveDischargeReq_flg>"
  [BOUTP_outputs] -> bus_selector/1
  Ground/1 -> OR/2
  Ground1/1 -> OR/3
  detect_change1/1 -> OR/4
  bus_selector1/1 -> detect_change1/1  "<VOUTP_DCDCEnaReq_flg>"
  [BOUTP_outputs] -> bus_selector1/1
  detect_change2/1 -> OR/5
  Data Type Conversion1/1 -> detect_change2/1
  convert_out/1 -> Data Type Conversion1/1
  bus_selector2/1 -> convert_out/1  "<VOUTP_DCDCVoltSetpoint_V>"
  [BOUTP_outputs] -> bus_selector2/1
  Ground2/1 -> OR/6
  Ground3/1 -> OR/7
  Ground4/1 -> OR/8
  detect_change3/1 -> OR/9
  bus_selector3/1 -> detect_change3/1  "<VOUTP_FrActvDmpDisabReq_flg>"
  [BOUTP_outputs] -> bus_selector3/1
  detect_change4/1 -> OR/10
  bus_selector4/1 -> detect_change4/1  "<VOUTP_FrMCUEnaReq_flg>"
  [BOUTP_outputs] -> bus_selector4/1
  detect_change5/1 -> OR/11
  bus_selector5/1 -> detect_change5/1  "<VOUTP_HVBatCnctReq_flg>"
  [BOUTP_outputs] -> bus_selector5/1
  detect_change6/1 -> OR/12
  bus_selector6/1 -> detect_change6/1  "<VOUTP_HVSysReadyToCharge_enum>"
  [BOUTP_outputs] -> bus_selector6/1
  Ground5/1 -> OR/13
  detect_change7/1 -> OR/14
  bus_selector7/1 -> detect_change7/1  "<VOUTP_MSACtrlSta_enum>"
  [BOUTP_outputs] -> bus_selector7/1
  detect_change8/1 -> OR/15
  bus_selector8/1 -> detect_change8/1  "<VOUTP_ActParkRequest_flg>"
  [BOUTP_outputs] -> bus_selector8/1
  detect_change9/1 -> OR/16
  bus_selector9/1 -> detect_change9/1  "<VOUTP_PowerSta_enum>"
  [BOUTP_outputs] -> bus_selector9/1
  Ground6/1 -> OR/17
  detect_change10/1 -> OR/18
  bus_selector10/1 -> detect_change10/1  "<VOUTP_RrActvDmpDisabReq_flg>"
  [BOUTP_outputs] -> bus_selector10/1
  detect_change11/1 -> OR/19
  bus_selector11/1 -> detect_change11/1  "<VOUTP_RrMCUEnaReq_flg>"
  [BOUTP_outputs] -> bus_selector11/1
  detect_change12/1 -> OR/20
  bus_selector12/1 -> detect_change12/1  "<VOUTP_ShiftGearPosn_enum>"
  [BOUTP_outputs] -> bus_selector12/1

== system halout/HAL_OUT/CAN3/FD_VCU2_0x154 ==
  BSCP_outputs : Inport  OutDataTypeStr=Bus: BSCP_outputs
  BOUTP_outputs : Inport  Port=2  OutDataTypeStr=Bus: BOUTP_outputs
  Trigger : TriggerPort  TriggerType=function-call  VariantControl=(inherit)
  Byte_0 : Subsystem
  Byte_1 : Subsystem
  Byte_10 : Subsystem
  Byte_11 : Subsystem
  Byte_12 : Subsystem
  Byte_13 : Subsystem
  Byte_14 : Subsystem
  Byte_15 : Subsystem
  Byte_16 : Subsystem
  Byte_17 : Subsystem
  Byte_18 : Subsystem
  Byte_19 : Subsystem
  Byte_2 : Subsystem
  Byte_20 : Subsystem
  Byte_21 : Subsystem
  Byte_22 : Subsystem
  Byte_23 : Subsystem
  Byte_3 : Subsystem
  Byte_4 : Subsystem
  Byte_5 : Subsystem
  Byte_6 : Subsystem
  Byte_7 : Subsystem
  Byte_8 : Subsystem
  Byte_9 : Subsystem
  CRC8_IfAction_Tx : FVT_lib/hal/CRC8_IfAction_Tx
  CSVCU2CAN1 : Subsystem
  Constant : Constant  Value=KHAL_CAN3FDVCU2E2E_flg
  Constant1 : Constant  Value=0x41
  Constant2 : Constant  Value=0x14
  Constant3 : Constant  Value=KHAL_CAN3FDVCU2E2E_flg
  Constant4 : Constant  Value=KHAL_CAN3FDVCU2E2E_flg
  FrIdcMax : Subsystem
  FrIdcMin : Subsystem
  FrTMTqReq : Subsystem
  FrTorqMax : Subsystem
  FrTorqMin : Subsystem
  FrUdcMax : Subsystem
  FrUdcMin : Subsystem
  Ground{,1..12} (13 alike) : Ground
  Mux2 : Mux  Inputs=23
  RCVCU2CAN1 : Subsystem
  RollingCounter_IfAction : FVT_lib/hal/RollingCounter_IfAction
  RollingCounter_IfAction1 : FVT_lib/hal/RollingCounter_IfAction
  RrIdcMax : Subsystem
  RrIdcMin : Subsystem
  RrTMTqReq : Subsystem
  RrTorqMax : Subsystem
  RrTorqMin : Subsystem
  RrUdcMax : Subsystem
  RrUdcMin : Subsystem
  Terminator : Terminator
  bus_creator : BusCreator  Inputs=16  OutDataTypeStr=Bus: DT_CAN3_SG_FD_VCU2  NonVirtualBus=on
  bus_selector : BusSelector  OutputSignals=VOUTP_RrIdcMax_A
  bus_selector1 : BusSelector  OutputSignals=VOUTP_RrIdcMax_A
  bus_selector10 : BusSelector  OutputSignals=VOUTP_FrUdcMin_V
  bus_selector11 : BusSelector  OutputSignals=VOUTP_FrUdcMin_V
  bus_selector12 : BusSelector  OutputSignals=VOUTP_RrTMTqReq_Nm
  bus_selector13 : BusSelector  OutputSignals=VOUTP_RrTMTqReq_Nm
  bus_selector14 : BusSelector  OutputSignals=VOUTP_FrTMTqReq_Nm
  bus_selector15 : BusSelector  OutputSignals=VOUTP_FrTMTqReq_Nm
  bus_selector16 : BusSelector  OutputSignals=VOUTP_FrIdcMax_A
  bus_selector17 : BusSelector  OutputSignals=VOUTP_FrIdcMax_A
  bus_selector18 : BusSelector  OutputSignals=VOUTP_FrIdcMin_A
  bus_selector19 : BusSelector  OutputSignals=VOUTP_FrIdcMin_A
  bus_selector2 : BusSelector  OutputSignals=VOUTP_RrIdcMin_A
  bus_selector20 : BusSelector  OutputSignals=VOUTP_FrIdcMax_A
  bus_selector21 : BusSelector  OutputSignals=VOUTP_FrIdcMin_A
  bus_selector22 : BusSelector  OutputSignals=VOUTP_FrTMTqReq_Nm
  bus_selector23 : BusSelector  OutputSignals=VOUTP_FrUdcMax_V
  bus_selector24 : BusSelector  OutputSignals=VOUTP_FrUdcMin_V
  bus_selector25 : BusSelector  OutputSignals=VOUTP_RrIdcMax_A
  bus_selector26 : BusSelector  OutputSignals=VOUTP_RrIdcMin_A
  bus_selector27 : BusSelector  OutputSignals=VOUTP_RrTMTqReq_Nm
  bus_selector28 : BusSelector  OutputSignals=VOUTP_RrUdcMax_V
  bus_selector29 : BusSelector  OutputSignals=VOUTP_RrUdcMin_V
  bus_selector3 : BusSelector  OutputSignals=VOUTP_RrIdcMin_A
  bus_selector4 : BusSelector  OutputSignals=VOUTP_RrUdcMax_V
  bus_selector5 : BusSelector  OutputSignals=VOUTP_RrUdcMax_V
  bus_selector6 : BusSelector  OutputSignals=VOUTP_RrUdcMin_V
  bus_selector7 : BusSelector  OutputSignals=VOUTP_RrUdcMin_V
  bus_selector8 : BusSelector  OutputSignals=VOUTP_FrUdcMax_V
  bus_selector9 : BusSelector  OutputSignals=VOUTP_FrUdcMax_V
  FD_VCU2 : Outport
  wires:
  BSCP_outputs/1 -> [BSCP_outputs]
  BOUTP_outputs/1 -> [BOUTP_outputs]
  [CAN3_CS_VCU2_CAN1] -> bus_creator/1  "CAN3_CS_VCU2_CAN1"
  [CAN3_Fr_IdcMax] -> bus_creator/2  "CAN3_Fr_IdcMax"
  [CAN3_Fr_IdcMin] -> bus_creator/3  "CAN3_Fr_IdcMin"
  [CAN3_Fr_TMTqReq] -> bus_creator/4  "CAN3_Fr_TMTqReq"
  [CAN3_Fr_TorqMax] -> bus_creator/5  "CAN3_Fr_TorqMax"
  [CAN3_Fr_TorqMin] -> bus_creator/6  "CAN3_Fr_TorqMin"
  [CAN3_Fr_UdcMax] -> bus_creator/7  "CAN3_Fr_UdcMax"
  [CAN3_Fr_UdcMin] -> bus_creator/8  "CAN3_Fr_UdcMin"
  [CAN3_RC_VCU2_CAN1] -> bus_creator/9  "CAN3_RC_VCU2_CAN1"
  [CAN3_Rr_IdcMax] -> bus_creator/10  "CAN3_Rr_IdcMax"
  [CAN3_Rr_IdcMin] -> bus_creator/11  "CAN3_Rr_IdcMin"
  [CAN3_Rr_TMTqReq] -> bus_creator/12  "CAN3_Rr_TMTqReq"
  [CAN3_Rr_TorqMax] -> bus_creator/13  "CAN3_Rr_TorqMax"
  [CAN3_Rr_TorqMin] -> bus_creator/14  "CAN3_Rr_TorqMin"
  [CAN3_Rr_UdcMax] -> bus_creator/15  "CAN3_Rr_UdcMax"
  [CAN3_Rr_UdcMin] -> bus_creator/16  "CAN3_Rr_UdcMin"
  bus_creator/1 -> FD_VCU2/1
  CSVCU2CAN1/1(CAN3_CS_VCU2_CAN1) -> [CAN3_CS_VCU2_CAN1]
  FrIdcMax/1(CAN3_Fr_IdcMax) -> [CAN3_Fr_IdcMax]
  FrIdcMin/1(CAN3_Fr_IdcMin) -> [CAN3_Fr_IdcMin]
  FrTMTqReq/1(CAN3_Fr_TMTqReq) -> [CAN3_Fr_TMTqReq]
  FrTorqMax/1(CAN3_Fr_TorqMax) -> [CAN3_Fr_TorqMax]
  FrTorqMin/1(CAN3_Fr_TorqMin) -> [CAN3_Fr_TorqMin]
  FrUdcMax/1(CAN3_Fr_UdcMax) -> [CAN3_Fr_UdcMax]
  FrUdcMin/1(CAN3_Fr_UdcMin) -> [CAN3_Fr_UdcMin]
  RCVCU2CAN1/1(CAN3_RC_VCU2_CAN1) -> [CAN3_RC_VCU2_CAN1]
  RrIdcMax/1(CAN3_Rr_IdcMax) -> [CAN3_Rr_IdcMax]
  RrIdcMin/1(CAN3_Rr_IdcMin) -> [CAN3_Rr_IdcMin]
  RrTMTqReq/1(CAN3_Rr_TMTqReq) -> [CAN3_Rr_TMTqReq]
  RrTorqMax/1(CAN3_Rr_TorqMax) -> [CAN3_Rr_TorqMax]
  RrTorqMin/1(CAN3_Rr_TorqMin) -> [CAN3_Rr_TorqMin]
  RrUdcMax/1(CAN3_Rr_UdcMax) -> [CAN3_Rr_UdcMax]
  RrUdcMin/1(CAN3_Rr_UdcMin) -> [CAN3_Rr_UdcMin]
  Byte_0/1(Byte_0) -> Terminator/1
  Byte_1/1(Byte_1) -> [Byte_1]
  Byte_2/1(Byte_2) -> [Byte_2]
  Byte_3/1(Byte_3) -> [Byte_3]
  Byte_4/1(Byte_4) -> [Byte_4]
  Byte_5/1(Byte_5) -> [Byte_5]
  Byte_6/1(Byte_6) -> [Byte_6]
  Byte_7/1(Byte_7) -> [Byte_7]
  Byte_8/1(Byte_8) -> [Byte_8]
  Byte_9/1(Byte_9) -> [Byte_9]
  Byte_10/1(Byte_10) -> [Byte_10]
  Byte_11/1(Byte_11) -> [Byte_11]
  Byte_12/1(Byte_12) -> [Byte_12]
  Byte_13/1(Byte_13) -> [Byte_13]
  Byte_14/1(Byte_14) -> [Byte_14]
  Byte_15/1(Byte_15) -> [Byte_15]
  Byte_16/1(Byte_16) -> [Byte_16]
  Byte_17/1(Byte_17) -> [Byte_17]
  Byte_18/1(Byte_18) -> [Byte_18]
  Byte_19/1(Byte_19) -> [Byte_19]
  Byte_20/1(Byte_20) -> [Byte_20]
  Byte_21/1(Byte_21) -> [Byte_21]
  Byte_22/1(Byte_22) -> [Byte_22]
  Byte_23/1(Byte_23) -> [Byte_23]
  Mux2/1 -> CRC8_IfAction_Tx/4
  Constant/1 -> CRC8_IfAction_Tx/1
  Constant1/1 -> CRC8_IfAction_Tx/2
  Constant2/1 -> CRC8_IfAction_Tx/3
  CRC8_IfAction_Tx/1 -> [CS_VCU2_CAN1]
  Ground/1 -> Byte_0/1(CS_VCU2_CAN1)
  [Byte_1] -> Mux2/1
  RollingCounter_IfAction/1 -> Byte_1/1(RC_VCU2_CAN1)
  Constant3/1 -> RollingCounter_IfAction/1
  [Byte_2] -> Mux2/2
  bus_selector/1 -> Byte_2/1(Rr_IdcMax)  "<VOUTP_RrIdcMax_A>"
  [BOUTP_outputs] -> bus_selector/1
  [Byte_3] -> Mux2/3
  bus_selector1/1 -> Byte_3/1(Rr_IdcMax)  "<VOUTP_RrIdcMax_A>"
  [BOUTP_outputs] -> bus_selector1/1
  bus_selector2/1 -> Byte_3/2(Rr_IdcMin)  "<VOUTP_RrIdcMin_A>"
  [BOUTP_outputs] -> bus_selector2/1
  [Byte_4] -> Mux2/4
  bus_selector3/1 -> Byte_4/1(Rr_IdcMin)  "<VOUTP_RrIdcMin_A>"
  [BOUTP_outputs] -> bus_selector3/1
  [Byte_5] -> Mux2/5
  Ground1/1 -> Byte_5/1(Rr_TorqMax)
  [Byte_6] -> Mux2/6
  Ground2/1 -> Byte_6/1(Rr_TorqMax)
  Ground3/1 -> Byte_6/2(Rr_TorqMin)
  [Byte_7] -> Mux2/7
  Ground4/1 -> Byte_7/1(Rr_TorqMin)
  [Byte_8] -> Mux2/8
  bus_selector4/1 -> Byte_8/1(Rr_UdcMax)  "<VOUTP_RrUdcMax_V>"
  [BOUTP_outputs] -> bus_selector4/1
  [Byte_9] -> Mux2/9
  bus_selector5/1 -> Byte_9/1(Rr_UdcMax)  "<VOUTP_RrUdcMax_V>"
  [BOUTP_outputs] -> bus_selector5/1
  bus_selector6/1 -> Byte_9/2(Rr_UdcMin)  "<VOUTP_RrUdcMin_V>"
  [BOUTP_outputs] -> bus_selector6/1
  [Byte_10] -> Mux2/10
  bus_selector7/1 -> Byte_10/1(Rr_UdcMin)  "<VOUTP_RrUdcMin_V>"
  [BOUTP_outputs] -> bus_selector7/1
  [Byte_11] -> Mux2/11
  bus_selector8/1 -> Byte_11/1(Fr_UdcMax)  "<VOUTP_FrUdcMax_V>"
  [BOUTP_outputs] -> bus_selector8/1
  [Byte_12] -> Mux2/12
  bus_selector9/1 -> Byte_12/1(Fr_UdcMax)  "<VOUTP_FrUdcMax_V>"
  [BOUTP_outputs] -> bus_selector9/1
  bus_selector10/1 -> Byte_12/2(Fr_UdcMin)  "<VOUTP_FrUdcMin_V>"
  [BOUTP_outputs] -> bus_selector10/1
  [Byte_13] -> Mux2/13
  bus_selector11/1 -> Byte_13/1(Fr_UdcMin)  "<VOUTP_FrUdcMin_V>"
  [BOUTP_outputs] -> bus_selector11/1
  [Byte_14] -> Mux2/14
  bus_selector12/1 -> Byte_14/1(Rr_TMTqReq)  "<VOUTP_RrTMTqReq_Nm>"
  [BOUTP_outputs] -> bus_selector12/1
  [Byte_15] -> Mux2/15
  bus_selector13/1 -> Byte_15/1(Rr_TMTqReq)  "<VOUTP_RrTMTqReq_Nm>"
  [BOUTP_outputs] -> bus_selector13/1
  [Byte_16] -> Mux2/16
  bus_selector14/1 -> Byte_16/1(Fr_TMTqReq)  "<VOUTP_FrTMTqReq_Nm>"
  [BOUTP_outputs] -> bus_selector14/1
  [Byte_17] -> Mux2/17
  bus_selector15/1 -> Byte_17/1(Fr_TMTqReq)  "<VOUTP_FrTMTqReq_Nm>"
  [BOUTP_outputs] -> bus_selector15/1
  [Byte_18] -> Mux2/18
  bus_selector16/1 -> Byte_18/1(Fr_IdcMax)  "<VOUTP_FrIdcMax_A>"
  [BOUTP_outputs] -> bus_selector16/1
  [Byte_19] -> Mux2/19
  bus_selector17/1 -> Byte_19/1(Fr_IdcMax)  "<VOUTP_FrIdcMax_A>"
  [BOUTP_outputs] -> bus_selector17/1
  bus_selector18/1 -> Byte_19/2(Fr_IdcMin)  "<VOUTP_FrIdcMin_A>"
  [BOUTP_outputs] -> bus_selector18/1
  [Byte_20] -> Mux2/20
  bus_selector19/1 -> Byte_20/1(Fr_IdcMin)  "<VOUTP_FrIdcMin_A>"
  [BOUTP_outputs] -> bus_selector19/1
  [Byte_21] -> Mux2/21
  Ground5/1 -> Byte_21/1(Fr_TorqMax)
  [Byte_22] -> Mux2/22
  Ground6/1 -> Byte_22/1(Fr_TorqMax)
  Ground7/1 -> Byte_22/2(Fr_TorqMin)
  [Byte_23] -> Mux2/23
  Ground8/1 -> Byte_23/1(Fr_TorqMin)
  [CS_VCU2_CAN1] -> CSVCU2CAN1/1(CSVCU2CAN1)
  bus_selector20/1 -> FrIdcMax/1(FrIdcMax)  "<VOUTP_FrIdcMax_A>"
  [BOUTP_outputs] -> bus_selector20/1
  bus_selector21/1 -> FrIdcMin/1(FrIdcMin)  "<VOUTP_FrIdcMin_A>"
  [BOUTP_outputs] -> bus_selector21/1
  bus_selector22/1 -> FrTMTqReq/1(FrTMTqReq)  "<VOUTP_FrTMTqReq_Nm>"
  [BOUTP_outputs] -> bus_selector22/1
  Ground9/1 -> FrTorqMax/1(FrTorqMax)
  Ground10/1 -> FrTorqMin/1(FrTorqMin)
  bus_selector23/1 -> FrUdcMax/1(FrUdcMax)  "<VOUTP_FrUdcMax_V>"
  [BOUTP_outputs] -> bus_selector23/1
  bus_selector24/1 -> FrUdcMin/1(FrUdcMin)  "<VOUTP_FrUdcMin_V>"
  [BOUTP_outputs] -> bus_selector24/1
  RollingCounter_IfAction1/1 -> RCVCU2CAN1/1(RCVCU2CAN1)
  Constant4/1 -> RollingCounter_IfAction1/1
  bus_selector25/1 -> RrIdcMax/1(RrIdcMax)  "<VOUTP_RrIdcMax_A>"
  [BOUTP_outputs] -> bus_selector25/1
  bus_selector26/1 -> RrIdcMin/1(RrIdcMin)  "<VOUTP_RrIdcMin_A>"
  [BOUTP_outputs] -> bus_selector26/1
  bus_selector27/1 -> RrTMTqReq/1(RrTMTqReq)  "<VOUTP_RrTMTqReq_Nm>"
  [BOUTP_outputs] -> bus_selector27/1
  Ground11/1 -> RrTorqMax/1(RrTorqMax)
  Ground12/1 -> RrTorqMin/1(RrTorqMin)
  bus_selector28/1 -> RrUdcMax/1(RrUdcMax)  "<VOUTP_RrUdcMax_V>"
  [BOUTP_outputs] -> bus_selector28/1
  bus_selector29/1 -> RrUdcMin/1(RrUdcMin)  "<VOUTP_RrUdcMin_V>"
  [BOUTP_outputs] -> bus_selector29/1

== system halout/HAL_OUT/CAN3/FD_VCU2_Tx ==
  TxReq : Inport
  Chart : Stateflow chart  TreatAsAtomicUnit=on
  Constant : Constant  Value=C_TASK_5MS_S
  Constant3 : Constant  Value=CycleTime
  Data Type Conversion : DataTypeConversion  OutDataTypeStr=uint16
  Divide : Product  Inputs=*/
  Gain : Gain  Gain=0.001
  TxTrigger : Outport
  wires:
  Data Type Conversion/1 -> Chart/2(CycleCnt)
  Constant3/1 -> Gain/1
  Gain/1 -> Divide/1
  Chart/1(TxTrigger()) -> TxTrigger/1
  Divide/1 -> Data Type Conversion/1
  TxReq/1 -> Chart/1(TxReq)
  Constant/1 -> Divide/2
